simulink model "control_strategy_1"  (R2024b)
settings: Solver=VariableStepAuto  StartTime=0.0  StopTime=0.3  MaxStep=1e-3  MinStep=1e-9  RelTol=1e-3
values from neighbouring files (symbols this model uses):
  C_filtre = 1 / (Lc * (2 * pi * 2000)^2)    (= 2.53302959106e-06)    [acdc_converter_parameters.m]
  Ccb = 330e-6    (= 0.00033)    [dcdc_converter_parameters.m]
  Cdc = 2200e-6    (= 0.0022)    [acdc_converter_parameters.m]
  Ci = 220e-6    (= 0.00022)    [dcdc_converter_parameters.m]
  Is = P / Vac    [acdc_converter_parameters.m]
  KI = KP * Wci_out    [dcdc_converter_main.m]
  KI_curr_d = 2 * pi * w_i * rac    [acdc_converter_main.m]
  KI_curr_q = 2 * pi * w_i * rac    [acdc_converter_main.m]
  KI_q = C_q.Ki    [acdc_converter_main.m]
  KI_volt = C_volt.Ki    [acdc_converter_main.m]
  KP = Wbi_dc / (DCGain_iod * Wci_out)    [dcdc_converter_main.m]
  KP_curr_d = 2 * pi * w_i * Lc    [acdc_converter_main.m]
  KP_curr_q = 2 * pi * w_i * Lc    [acdc_converter_main.m]
  KP_q = C_q.Kp    [acdc_converter_main.m]
  KP_volt = C_volt.Kp    [acdc_converter_main.m]
  Lb = 3e-3    (= 0.003)    [dcdc_converter_parameters.m]
  Lc = 2.5e-3    (= 0.0025)    [acdc_converter_parameters.m]
  Lsi = 105e-6    (= 0.000105)    [dcdc_converter_parameters.m]
  P = 500    [main_control_strategy_1.m]
  phase = 0    [acdc_converter_parameters.m]
  Q = 0    [main_control_strategy_1.m]
  rac = 1e-3    (= 0.001)    [acdc_converter_parameters.m]
  rb = 1e-3    (= 0.001)    [dcdc_converter_parameters.m]
  ro = 270e-3    (= 0.27)    [dcdc_converter_parameters.m]
  rsi = 1e-3    (= 0.001)    [dcdc_converter_parameters.m]
  Vac = 120    [acdc_converter_parameters.m]
  Vb = 48    [dcdc_converter_parameters.m]
  Vdc0 = Vdc    (= 200)    [acdc_converter_parameters.m]
  Vs0 = Vac    (= 120)    [acdc_converter_parameters.m]
  w = 2 * pi * f    (= 376.991118431)    [acdc_converter_parameters.m]
  Zl = w * Lc    (= 0.942477796077)    [acdc_converter_parameters.m]
undefined symbols (not defined in the file or in its folder): q_switch
libraries: spsSeriesRLCBranchLib x6, spsMosfetLib x6, slpidlib x5, spsVoltageMeasurementLib x4, spsMeanLib x4, spsParallelRLCBranchLib x3, spsCurrentMeasurementLib x3, spsTHDLib x3, spsACVoltageSourceLib x1, spsGroundLib x1, spsPWMGenerator2LevelLib x1, eePowerMeasurement x1
settings Model: Creator=casti  LastModifiedBy=Asus
settings OptimizationCC: ReuseModelBlockBuffer=off
settings RTWCC: GPUComputeCapability=3.5

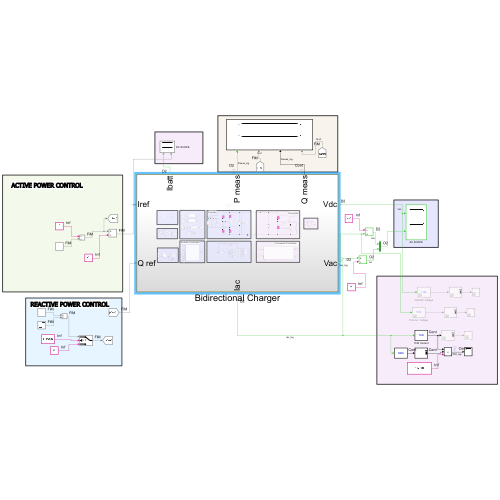
[thumbnail: Simulink's stored preview of the top-level diagram]
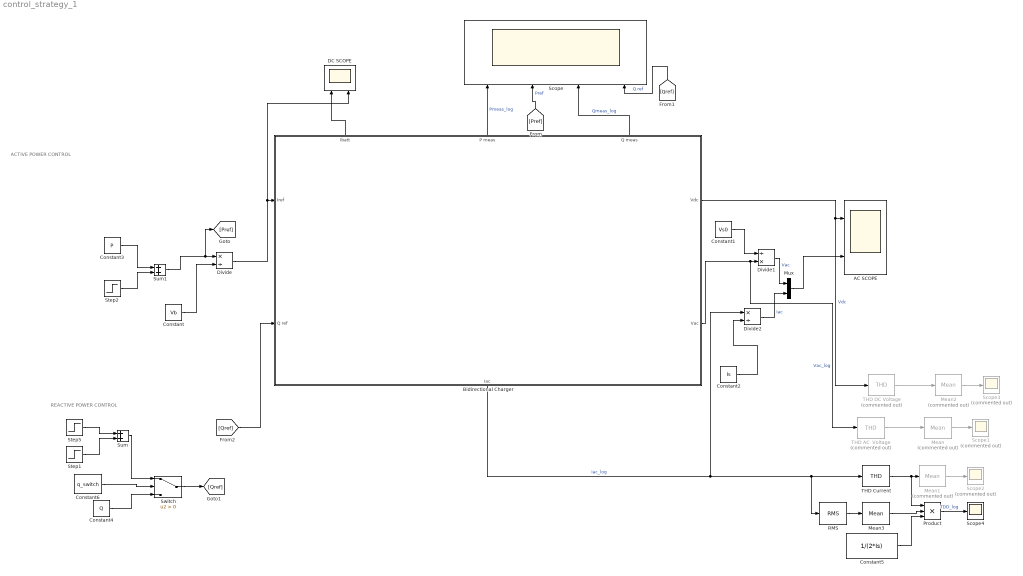
== system control_strategy_1 ==
  note: ACTIVE POWER CONTROL
  note: REACTIVE POWER CONTROL
  AC SCOPE : Scope  NumInputPorts=2
  Bidirectional Charger : Subsystem
      settings: PortSchema="{\"entries\":[{\"content\":{\"sides\":[{\"content\":{\"connectorIds\":[\"In1\",\"In2\"]},\"type\":\"ConnectorPlacement.EquallySpacedRectSide\",\"uuid\":\"0e8ef780-485e-4c8b-9a8b-f034f795c892\"},{\"content\":{\"connectorIds\":[\"Out1\",\"Out2\"],\"side\":\"RIGHT\"},\"type\":\"ConnectorPlacement.EquallySpacedRectSide\",\"uuid\":\"9fd702af-2122-4ac4-9fd2-64e19671b5dd\"},{\"content\":{\"connectorIds\":[\"Out4\",\"Out5\",\"Out6\"],\"side\":\"TOP\"},\"type\":\"ConnectorPlacement.EquallySpacedRectSide\",\"uuid\":\"331bdb16-1cb1-49e4-96bf-e66e7b38baa0\"},{\"content\":{\"connectorIds\":[\"Out3\"],\"side\":\"BOTTOM\"},\"type\":\"ConnectorPlacement.EquallySpacedRectSide\",\"uuid\":\"d0f2bc9b-30cd-4241-b923-1d5d9998130d\"}]},\"type\":\"ConnectorPlacement.EquallySpacedConnector\",\"uuid\":\"78325ce0-b63a-4b2a-b520-d47ca5f2449f\"}],\"packageUris\":[\"http://schema.mathworks.com/mf0/Connector/R2020b\"],\"version\":\"1.0\"}"
  Constant : Constant  Value=Vb
  Constant1 : Constant  Value=Vs0
  Constant2 : Constant  Value=Is
  Constant3 : Constant  Value=P
  Constant4 : Constant  Value=Q
  Constant5 : Constant  Value=1/(2*Is)
  Constant6 : Constant  Value=q_switch
  DC SCOPE : Scope  NumInputPorts=2
  Divide : Product  Inputs=*/
  Divide1 : Product  Inputs=/*
  Divide2 : Product  Inputs=*/
  Mean : spsMeanLib/Mean  Commented=on  Freq=60  Vinit=0  Ts=0
  Mean1 : spsMeanLib/Mean  Commented=on  Freq=60  Vinit=0  Ts=0
  Mean2 : spsMeanLib/Mean  Commented=on  Freq=120  Vinit=0  Ts=0
  Mean3 : spsMeanLib/Mean  Freq=60  Vinit=0  Ts=0
  Mux : Mux  Inputs=2
  Product : Product  Inputs=3
  RMS : spsRMSLib/RMS  TrueRMS=on  Freq=60  RMSInit=120  Ts=0
  Scope : Scope  NumInputPorts=4
  Scope1 : Scope  Commented=on
  Scope2 : Scope  Commented=on
  Scope3 : Scope  Commented=on
  Scope4 : Scope
  Step1 : Step  Time=10  After=-2*Q  SampleTime=0
  Step2 : Step  Time=10  After=-2*P  SampleTime=0
  Step5 : Step  Time=0.05  After=Q  SampleTime=0
  Sum : Sum
  Sum1 : Sum
  Switch : Switch  Criteria=u2 > Threshold  SaturateOnIntegerOverflow=off  InputSameDT=off
  THD AC  Voltage : spsTHDLib/THD  Commented=on  Freq=60  Ts=0
  THD Current : spsTHDLib/THD  Freq=60  Ts=0
  THD DC Voltage : spsTHDLib/THD  Commented=on  Freq=120  Ts=0
  wires:
  Constant/1 -> Divide/2
  Divide/1 -> DC SCOPE/2, Bidirectional Charger/1(Iref)
  Bidirectional Charger/4(Ibatt) -> DC SCOPE/1
  Bidirectional Charger/1(Vdc) -> THD DC Voltage/1, AC SCOPE/1  "Vdc"
  Bidirectional Charger/5(P meas) -> Scope/1  "Pmeas_log"
  Bidirectional Charger/6(Q meas) -> Scope/3  "Qmeas_log"
  [Pref] -> Scope/2  "Pref"
  [Qref] -> Scope/4  "Q ref"
  Mux/1 -> AC SCOPE/2
  Bidirectional Charger/2(Vac) -> THD AC  Voltage/1, Divide1/2  "Vac_log"
  Constant1/1 -> Divide1/1
  Constant2/1 -> Divide2/2
  Divide2/1 -> Mux/2  "Iac"
  Divide1/1 -> Mux/1  "Vac"
  Mean/1 -> Scope1/1
  THD AC  Voltage/1 -> Mean/1
  Mean1/1 -> Scope2/1
  THD Current/1 -> Product/1, Mean1/1
  THD DC Voltage/1 -> Mean2/1
  Mean2/1 -> Scope3/1
  [Qref] -> Bidirectional Charger/2(Q ref)
  RMS/1 -> Mean3/1
  Constant5/1 -> Product/3
  Product/1 -> Scope4/1  "TDD_log"
  Mean3/1 -> Product/2
  Bidirectional Charger/3(Iac) -> RMS/1, THD Current/1, Divide2/1  "Iac_log"
  Constant4/1 -> Switch/3
  Switch/1 -> [Qref]
  Constant6/1 -> Switch/2
  Step5/1 -> Sum/1
  Sum/1 -> Switch/1
  Step1/1 -> Sum/2
  Step2/1 -> Sum1/2
  Constant3/1 -> Sum1/1
  Sum1/1 -> [Pref], Divide/1

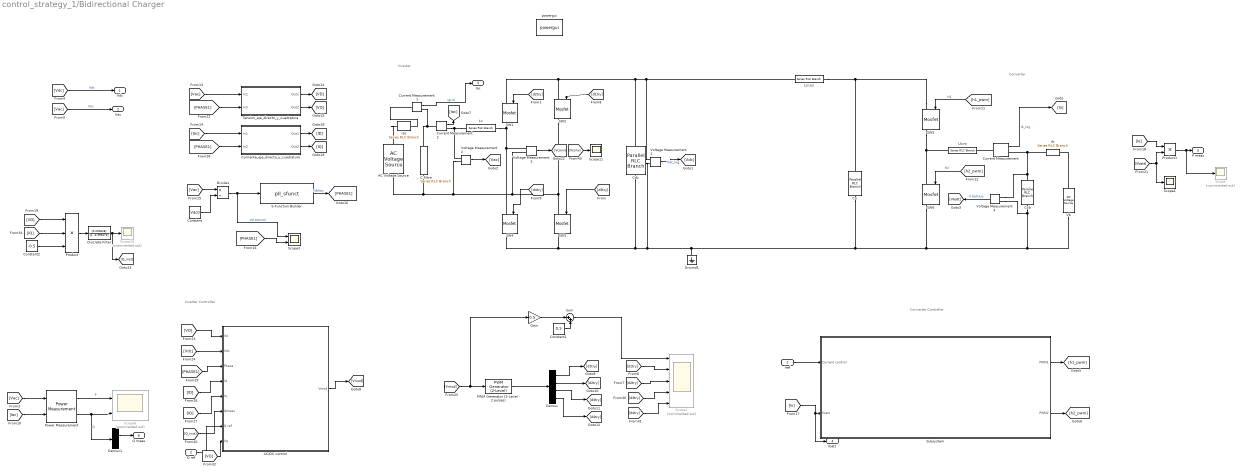
== system control_strategy_1/Bidirectional Charger ==
  note: Converter
  note: Inverter Controller
  note: Inverter
  note: Converter Controller
  Iref : Inport
  Q ref : Inport  Port=2
  AC Voltage Source : spsACVoltageSourceLib/AC Voltage Source  Amplitude=Vac*sqrt(2)  Phase=0  Frequency=60  SampleTime=0  Measurements=None  BusType=swing  Pref=10e3  Qref=0  Qmin=-inf  Qmax=+inf
  AC/DC control : Subsystem
  C filtre : spsSeriesRLCBranchLib/Series RLC Branch  LConnTagsString=__new0  RConnTagsString=__new0  BranchType=C  Resistance=rac  Inductance=Lc  SetiL0=off  InitialCurrent=Io0  Capacitance=C_filtre  Setx0=off  InitialVoltage=0  Measurements=None
  Ccb : spsParallelRLCBranchLib/Parallel RLC Branch  LConnTagsString=a  RConnTagsString=__new0  BranchType=C  Resistance=1  Inductance=1e-3  SetiL0=off  InitialCurrent=0  Capacitance=Ccb  Setx0=on  InitialVoltage=Vb  Measurements=None
  Cdc : spsParallelRLCBranchLib/Parallel RLC Branch  LConnTagsString=a  RConnTagsString=__new0  BranchType=C  Resistance=1  Inductance=1e-3  SetiL0=off  InitialCurrent=0  Capacitance=Cdc  Setx0=on  InitialVoltage=Vdc  Measurements=None
  Constant : Constant  Value=Vdc0
  Constant1 : Constant  Value=0.5
  Constant2 : Constant  Value=-0.5
  Corriente_eje_directo_y_cuadratura : Subsystem
  Csi : spsParallelRLCBranchLib/Parallel RLC Branch  LConnTagsString=a  RConnTagsString=__new0  BranchType=C  Resistance=1  Inductance=1e-3  SetiL0=off  InitialCurrent=0  Capacitance=Ci  Setx0=on  InitialVoltage=Vdc  Measurements=None
  Current Measurement : spsCurrentMeasurementLib/Current Measurement  PhasorSimulation=off  OutputType=Complex  PSBequivalent=0
  Current Measurement1 : spsCurrentMeasurementLib/Current Measurement  PhasorSimulation=off  OutputType=Complex  PSBequivalent=0
  Current Measurement2 : spsCurrentMeasurementLib/Current Measurement  PhasorSimulation=off  OutputType=Complex  PSBequivalent=0
  Demux : Demux
  Demux1 : Demux
  Discrete Filter : DiscreteFilter  Numerator=[0.000628]  Denominator=[1 -0.999372]
  Divide1 : Product  Inputs=*/
  Gain : Gain  Gain=0.5
  Ground1 : spsGroundLib/Ground  LConnTagsString=a
  Lb,ro : spsSeriesRLCBranchLib/Series RLC Branch  LConnTagsString=__new0  RConnTagsString=__new0  BranchType=RL  Resistance=ro  Inductance=Lb  SetiL0=off  InitialCurrent=Io0  Capacitance=1e-6  Setx0=off  InitialVoltage=0  Measurements=None
  Lc : spsSeriesRLCBranchLib/Series RLC Branch  LConnTagsString=__new0  RConnTagsString=__new0  BranchType=L  Resistance=rac  Inductance=Lc  SetiL0=off  InitialCurrent=Io0  Capacitance=1e-6  Setx0=off  InitialVoltage=0  Measurements=None
  Lsi,rsi : spsSeriesRLCBranchLib/Series RLC Branch  LConnTagsString=__new0  RConnTagsString=__new0  BranchType=RL  Resistance=rsi  Inductance=Lsi  SetiL0=off  InitialCurrent=Io0  Capacitance=1e-6  Setx0=off  InitialVoltage=0  Measurements=None
  PWM Generator (2-Level - 2 pulses) : spsPWMGenerator2LevelLib/PWM Generator (2-Level)  ModulatorType=Single-phase full-bridge - Bipolar modulation (4 pulses)  ModulatorMode=Unsynchronized  Fc=20000  Pc=90  nF=27  MinMax="[ -1  1 ]"  SamplingTechnique=Natural  ModulatingSignals=off  m=0.6  Freq=60  Phase=30  Ts=5e-6  ShowCarrierOutport=off
  Power Measurement : eePowerMeasurement/Power Measurement  LabelModeActiveChoice=Continuous  F=60  K=[0 1 2 3]  Ts=0
  Product : Product  Inputs=3
  Product1 : Product
  S-Function Builder : S-Function  FunctionName=pll_sfunct  SFunctionModules=pll_sfunct_wrapper.c  SFunctionDeploymentMode=off  EnableBusSupport=off  mask(S-Function Builder){}
      mask help: Simulink:masks:SFunctionBuilder_MD
      mask init:
      | val = [[.9  0.75 0.75 1 1 .9 .9 1]',[1 1 0.75 0.75 .9 .9 1 .9]'];try , sys = get_param(gcb,'SfunBuilderFcnName');if isempty(sys), sys = get_param(gcb,'FunctionName'); end,catch, sys = get_param(gcb,'FunctionName'); end
      settings: CopyFcn=set_param(gcbh,'LinkStatus','none')  OpenFcn=sfunctionwizard(gcbh)
      mask Display:
      | plot(val(:,1),val(:,2))
      | disp(sys)
      | port_label('input',1,sprintf('%s', 'Vac'),'interpreter','tex')
      | port_label('output',1,sprintf('%s', 'phase'),'interpreter','tex')
  SW{1..6} (6 alike) : spsMosfetLib/Mosfet  Ron=1e-3  Lon=0  Rd=0.00001  Vfd=0  IC=0  Rs=1e5  Cs=inf  Measurements=on
  Scope : Scope  Commented=on
  Scope1 : Scope
  Scope10 : Scope  Commented=on
  Scope11 : Scope
  Scope2 : Scope  Commented=on  NumInputPorts=5
  Scope3 : Scope  NumInputPorts=2
  Scope8 : Scope  Commented=on  NumInputPorts=2
  Subsystem : Subsystem
  Sum : Sum  Inputs=|++
  Tension_eje_directo_y_cuadratura : Subsystem
  Vb : spsDCVoltageSourceLib/DC Voltage Source  Amplitude=Vb  Measurements=None
  Voltage Measurement{1..4} (4 alike) : spsVoltageMeasurementLib/Voltage Measurement  PhasorSimulation=off  OutputType=Complex  PSBequivalent=0
  powergui : spspowerguiLib/powergui  Priority=1  SimulationMode=Discrete  SampleTime=5e-6  frequency=60  Iterations=50  frequencyindice=0  Pbase=100e6  ErrMax=1e-4  UnitsV=kV  UnitsW=MW  buscounter=0  FunctionMessages=off  echomessages=off  EnableUseOfTLC=off  CurrentSourceSwitches=off  DisableSnubberDevices=off  DisableRonSwitches=off  DisableVfSwitches=off  DisplayEquations=off  AutomaticDiscreteSolvers=off  SolverType=Tustin/Backward Euler (TBE)  Interpol=off  ExternalGateDelay=off  methode=off  Ts=100  x0status=blocks  SPID=on  SwTol=0  HookPort=off  NonlinearTolerance=1e-4  nMaxIteration=100  ContinueOnMaxIteration=off  RestoreLinks=warning  ResistiveCurrentMeasurement=off  Frange=[0:2:500]  Ylog=off  Xlog=on  ShowGrid=off  save=off  variable=ZData  structure=0  ZoomFFT=off  StartTime=0.0  cycles=1  DisplayStyle=1  fundamental=60  FreqAxis=off  MaxFrequency=1000  frequencyindicesteady=1  RmsSteady=1  display=off
  rac : spsSeriesRLCBranchLib/Series RLC Branch  LConnTagsString=__new0  RConnTagsString=__new0  BranchType=R  Resistance=rac  Inductance=Lc  SetiL0=off  InitialCurrent=Io0  Capacitance=1e-6  Setx0=off  InitialVoltage=0  Measurements=None
  rb : spsSeriesRLCBranchLib/Series RLC Branch  LConnTagsString=__new0  RConnTagsString=__new0  BranchType=R  Resistance=rb  Inductance=1e-3  SetiL0=off  InitialCurrent=0  Capacitance=1e-6  Setx0=off  InitialVoltage=0  Measurements=None
  Vdc : Outport
  Vac : Outport  Port=2
  Iac : Outport  Port=3
  Ibatt : Outport  Port=4
  P meas : Outport  Port=5
  Q meas : Outport  Port=6
  wires:
  Iref/1 -> Subsystem/1(Current control)
  [d2try] -> Scope2/3
  Voltage Measurement3/1 -> [Vconv]
  PWM Generator (2-Level - 2 pulses)/1 -> Demux/1
  [Vconv] -> Scope11/1
  [Io] -> Ibatt/1, Subsystem/2(Ibatt)
  [PHASE1] -> Corriente_eje_directo_y_cuadratura/2(In2)
  [h1_pwm] -> SW5/1  "H1"
  [Vac] -> Vac/1  "Vac"
  [Vac] -> Divide1/1
  AC/DC control/1(Vmod) -> [Vmod]
  Tension_eje_directo_y_cuadratura/1(Out1) -> [VD]
  Gain/1 -> Sum/1
  [Iac] -> Corriente_eje_directo_y_cuadratura/1(In1)
  Divide1/1 -> Scope3/1, S-Function Builder/1  "Vd control"
  Sum/1 -> Scope2/1
  [h2_pwm] -> SW6/1  "H2"
  Current Measurement2/1 -> [Iac]
  Subsystem/2(PWM2) -> [h2_pwm]
  Voltage Measurement1/1 -> [Vdc]  "Vdc_log"
  Current Measurement/1 -> [Io]  "Ib_log"
  [d2try] -> SW1/1
  Demux/4 -> [d4try]
  Constant1/1 -> Sum/2
  [Vdc] -> Vdc/1  "Vdc"
  [d1try] -> SW2/1
  Constant/1 -> Divide1/2
  [d4try] -> Scope2/5
  [d3try] -> SW3/1
  S-Function Builder/1 -> [PHASE1]  "Vdelay"
  Voltage Measurement2/1 -> [Vac]
  Demux/1 -> [d1try]
  [Vmod] -> Gain/1, PWM Generator (2-Level - 2 pulses)/1
  [d4try] -> SW4/1
  Subsystem/1(PWM1) -> [h1_pwm]
  [Vac] -> Tension_eje_directo_y_cuadratura/1(In1)
  Tension_eje_directo_y_cuadratura/2(Out2) -> [VQ]
  Corriente_eje_directo_y_cuadratura/1(Out1) -> [ID]
  Corriente_eje_directo_y_cuadratura/2(Out2) -> [IQ]
  [PHASE1] -> Scope3/2
  [PHASE1] -> Tension_eje_directo_y_cuadratura/2(In2)
  [ID] -> AC/DC control/4(Id)
  Demux/2 -> [d2try]
  Demux/3 -> [d3try]
  [d3try] -> Scope2/4
  [d1try] -> Scope2/2
  [Vdc] -> AC/DC control/2(Vdc)
  [VD] -> AC/DC control/1(Vd)
  [IQ] -> AC/DC control/5(Iq)
  [PHASE1] -> AC/DC control/3(Phase)
  Power Measurement/2 -> Demux1/1, Scope8/2  "Q"
  [Iac] -> Power Measurement/2
  Demux1/2 -> Q meas/1
  Power Measurement/1 -> Scope8/1  "P"
  [Vac] -> Power Measurement/1
  [Q_inst] -> AC/DC control/6(Qmeas)
  [VD] -> Product/1
  Discrete Filter/1 -> [Q_inst], Scope10/1
  Product/1 -> Discrete Filter/1
  [IQ] -> Product/2
  Constant2/1 -> Product/3
  Q ref/1 -> AC/DC control/7(Q ref)
  Voltage Measurement4/1 -> [Vbatt]  "V battery"
  [Io] -> Product1/1
  [Vbatt] -> Scope1/1, Product1/2
  Product1/1 -> Scope/1, P meas/1
  Current Measurement1/1 -> Iac/1  "igrid"
  [VQ] -> AC/DC control/8(Vq)
  connections:
  SW4/LConn1 -- Lc/RConn1 -- SW1/RConn1 -- Voltage Measurement3/LConn1
  SW5/LConn1 -- Csi/LConn1 -- Lsi,rsi/LConn1
  SW2/LConn1 -- Cdc/LConn1 -- Voltage Measurement1/LConn1 -- Lsi,rsi/RConn1 -- SW1/LConn1
  SW6/RConn1 -- Voltage Measurement4/LConn2 -- Ccb/RConn1 -- Vb/LConn1 -- Csi/RConn1 -- Cdc/RConn1 -- SW3/RConn1 -- SW4/RConn1 -- Voltage Measurement1/LConn2 -- Ground1/LConn1
  Vb/RConn1 -- rb/RConn1
  SW5/RConn1 -- SW6/LConn1 -- Lb,ro/LConn1
  C filtre/LConn1 -- Current Measurement1/RConn1 -- Current Measurement2/LConn1
  Voltage Measurement2/LConn2 -- AC Voltage Source/LConn1 -- C filtre/RConn1 -- SW2/RConn1 -- SW3/LConn1 -- Voltage Measurement3/LConn2
  Ccb/LConn1 -- rb/LConn1 -- Current Measurement/RConn1 -- Voltage Measurement4/LConn1
  Current Measurement/LConn1 -- Lb,ro/RConn1
  Lc/LConn1 -- Current Measurement2/RConn1 -- Voltage Measurement2/LConn1
  rac/RConn1 -- AC Voltage Source/RConn1
  Current Measurement1/LConn1 -- rac/LConn1

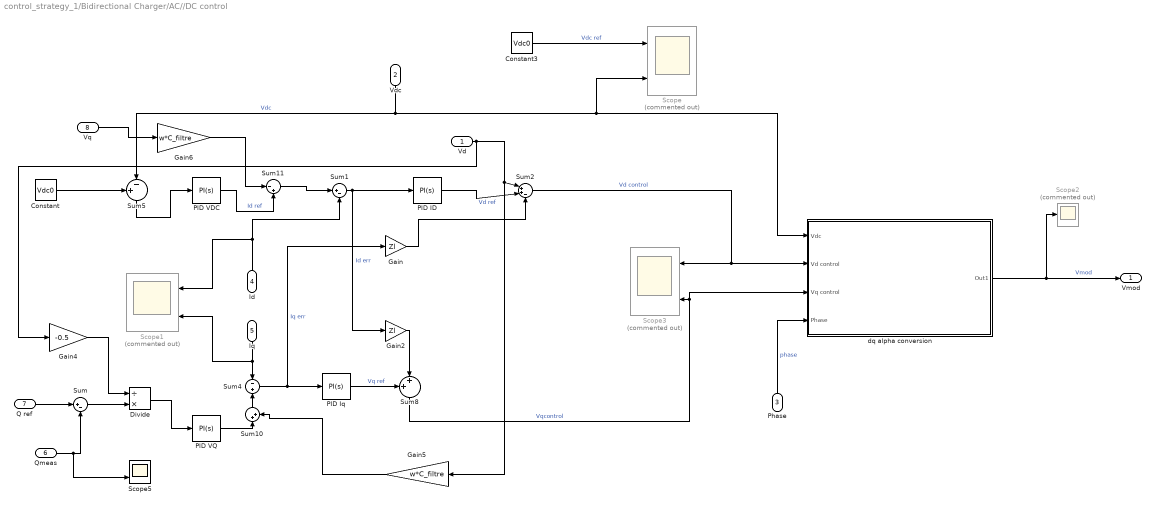
== system control_strategy_1/Bidirectional Charger/AC//DC control ==
  Vd : Inport
  Vdc : Inport  Port=2
  Phase : Inport  Port=3
  Id : Inport  Port=4
  Iq : Inport  Port=5
  Qmeas : Inport  Port=6
  Q ref : Inport  Port=7
  Vq : Inport  Port=8
  Constant : Constant  Value=Vdc0
  Constant3 : Constant  Value=Vdc0
  Divide : Product  Inputs=/*
  Gain : Gain  Gain=Zl
  Gain2 : Gain  Gain=Zl
  Gain4 : Gain  Gain=-0.5
  Gain5 : Gain  Gain=w*C_filtre
  Gain6 : Gain  Gain=w*C_filtre
  PID ID : slpidlib/PID Controller  Controller=PI  Form=Parallel  TimeDomain=Continuous-time  UseExternalTs=off  SampleTime=-1  IntegratorMethod=Forward Euler  FilterMethod=Forward Euler  ControllerParametersSource=internal  P=KP_curr_d  I=KI_curr_d  UseKiTs=off  D=0  UseExternalDerivativeSource=off  N=100  UseFilter=on  TunerSelectOption=Transfer Function Based (PID Tuner App)  InitialConditionSource=internal  InitialConditionForIntegrator=0  InitialConditionForFilter=0  DifferentiatorICPrevScaledInput=0  ExternalReset=none  TrackingMode=off  Kt=1  LimitOutput=off  SatLimitsSource=internal  UpperSaturationLimit=200  LowerSaturationLimit=-inf  LinearizeAsGain=on  AntiWindupMode=none  Kb=1  LimitIntegrator=off  UpperIntegratorSaturationLimit=inf  LowerIntegratorSaturationLimit=-inf  POutMin=[]  POutMax=[]  IOutMin=[]  IOutMax=[]  DOutMin=[]  DOutMax=[]  NOutMin=[]  NOutMax=[]  SumOutMin=[]  SumOutMax=[]  SaturationOutMin=[]  SaturationOutMax=[]  PParamMin=[]  PParamMax=[]  IParamMin=[]  IParamMax=[]  DParamMin=[]  DParamMax=[]  NParamMin=[]  NParamMax=[]  KbParamMin=[]  KbParamMax=[]  KtParamMin=[]  KtParamMax=[]  KbOutMin=[]  KbOutMax=[]  KtOutMin=[]  KtOutMax=[]  IntegratorOutMin=[]  IntegratorOutMax=[]  FilterOutMin=[]  FilterOutMax=[]  SumI1OutMin=[]  SumI1OutMax=[]  SumI2OutMin=[]  SumI2OutMax=[]  SumI3OutMin=[]  SumI3OutMax=[]  SumI4OutMin=[]  SumI4OutMax=[]  SumDOutMin=[]  SumDOutMax=[]  DifferentiatorOutMin=[]  DifferentiatorOutMax=[]  FilterDiffOutCoefMin=[]  FilterDiffOutCoefMax=[]  ReciprocalOutMin=[]  ReciprocalOutMax=[]  SumDenOutMin=[]  SumDenOutMax=[]  SumNumOutMin=[]  SumNumOutMax=[]  DivideOutMin=[]  DivideOutMax=[]  UdiffTsProdOutMin=[]  UdiffTsProdOutMax=[]  NTsProdOutMin=[]  NTsProdOutMax=[]  UintegralTsProdOutMin=[]  UintegralTsProdOutMax=[]  UngainTsProdOutMin=[]  UngainTsProdOutMax=[]  ClampingZeroOutDataTypeStr=Inherit: Inherit via back propagation  ClampingZeroOutMin=[]  ClampingZeroOutMax=[]  FilterDenConstantOutDataTypeStr=Inherit: Inherit via back propagation  FilterDenConstantOutMin=[]  FilterDenConstantOutMax=[]  PCopyOutDataTypeStr=Inherit: Inherit via back propagation  PCopyOutMin=[]  PCopyOutMax=[]  NCopyOutDataTypeStr=Inherit: Inherit via back propagation  NCopyOutMin=[]  NCopyOutMax=[]  IntegratorContinuousStateAttributes=''  IntegratorStateMustResolveToSignalObject=off  IntegratorRTWStateStorageClass=Auto  FilterContinuousStateAttributes=''  FilterStateMustResolveToSignalObject=off  FilterRTWStateStorageClass=Auto  ParallelPVariant=InternalParameters  IdealPVariant=Disabled  IVariant=InternalParameters  DVariant=Disabled  IntegratorVariant=Continuous  SatVariant=Disabled  AWVariant=Passthrough  PCopyVariant=Disabled  TRVariant=Disabled  FdbkBlocksVariant=Forward  IdealPFdbkVariant=Disabled  SatFdbkVariant=Disabled  DerivativeFilterVariant=Disabled  NVariant=Disabled  NCopyVariant=Disabled_SignalSpec  FilterICVariant=Disabled  IntegratorICVariant=InternalICs  ExternalResetVariant=Disabled  TRSumVariant=Passthrough  SumFdbkVariant=Disabled  SumVariant=Sum_PI  TsampFilterVariant=InternalTs  TsampNgainVariant=Passthrough  TsampIntegralVariant=Disabled_SignalSpec  ExternalSaturationOutDataTypeStr=Inherit: Same as second input  DerivativeSourceVariant=Disabled  PreIntVariant=InternalPreInt
  PID Iq : slpidlib/PID Controller  Controller=PI  Form=Parallel  TimeDomain=Continuous-time  UseExternalTs=off  SampleTime=-1  IntegratorMethod=Forward Euler  FilterMethod=Forward Euler  ControllerParametersSource=internal  P=KP_curr_q  I=KI_curr_q  UseKiTs=off  D=0  UseExternalDerivativeSource=off  N=100  UseFilter=on  TunerSelectOption=Transfer Function Based (PID Tuner App)  InitialConditionSource=internal  InitialConditionForIntegrator=0  InitialConditionForFilter=0  DifferentiatorICPrevScaledInput=0  ExternalReset=none  TrackingMode=off  Kt=1  LimitOutput=off  SatLimitsSource=internal  UpperSaturationLimit=15  LowerSaturationLimit=-15  LinearizeAsGain=on  AntiWindupMode=none  Kb=1  LimitIntegrator=off  UpperIntegratorSaturationLimit=inf  LowerIntegratorSaturationLimit=-inf  POutMin=[]  POutMax=[]  IOutMin=[]  IOutMax=[]  DOutMin=[]  DOutMax=[]  NOutMin=[]  NOutMax=[]  SumOutMin=[]  SumOutMax=[]  SaturationOutMin=[]  SaturationOutMax=[]  PParamMin=[]  PParamMax=[]  IParamMin=[]  IParamMax=[]  DParamMin=[]  DParamMax=[]  NParamMin=[]  NParamMax=[]  KbParamMin=[]  KbParamMax=[]  KtParamMin=[]  KtParamMax=[]  KbOutMin=[]  KbOutMax=[]  KtOutMin=[]  KtOutMax=[]  IntegratorOutMin=[]  IntegratorOutMax=[]  FilterOutMin=[]  FilterOutMax=[]  SumI1OutMin=[]  SumI1OutMax=[]  SumI2OutMin=[]  SumI2OutMax=[]  SumI3OutMin=[]  SumI3OutMax=[]  SumI4OutMin=[]  SumI4OutMax=[]  SumDOutMin=[]  SumDOutMax=[]  DifferentiatorOutMin=[]  DifferentiatorOutMax=[]  FilterDiffOutCoefMin=[]  FilterDiffOutCoefMax=[]  ReciprocalOutMin=[]  ReciprocalOutMax=[]  SumDenOutMin=[]  SumDenOutMax=[]  SumNumOutMin=[]  SumNumOutMax=[]  DivideOutMin=[]  DivideOutMax=[]  UdiffTsProdOutMin=[]  UdiffTsProdOutMax=[]  NTsProdOutMin=[]  NTsProdOutMax=[]  UintegralTsProdOutMin=[]  UintegralTsProdOutMax=[]  UngainTsProdOutMin=[]  UngainTsProdOutMax=[]  ClampingZeroOutDataTypeStr=Inherit: Inherit via back propagation  ClampingZeroOutMin=[]  ClampingZeroOutMax=[]  FilterDenConstantOutDataTypeStr=Inherit: Inherit via back propagation  FilterDenConstantOutMin=[]  FilterDenConstantOutMax=[]  PCopyOutDataTypeStr=Inherit: Inherit via back propagation  PCopyOutMin=[]  PCopyOutMax=[]  NCopyOutDataTypeStr=Inherit: Inherit via back propagation  NCopyOutMin=[]  NCopyOutMax=[]  IntegratorContinuousStateAttributes=''  IntegratorStateMustResolveToSignalObject=off  IntegratorRTWStateStorageClass=Auto  FilterContinuousStateAttributes=''  FilterStateMustResolveToSignalObject=off  FilterRTWStateStorageClass=Auto  ParallelPVariant=InternalParameters  IdealPVariant=Disabled  IVariant=InternalParameters  DVariant=Disabled  IntegratorVariant=Continuous  SatVariant=Disabled  AWVariant=Passthrough  PCopyVariant=Disabled  TRVariant=Disabled  FdbkBlocksVariant=Forward  IdealPFdbkVariant=Disabled  SatFdbkVariant=Disabled  DerivativeFilterVariant=Disabled  NVariant=Disabled  NCopyVariant=Disabled_SignalSpec  FilterICVariant=Disabled  IntegratorICVariant=InternalICs  ExternalResetVariant=Disabled  TRSumVariant=Passthrough  SumFdbkVariant=Disabled  SumVariant=Sum_PI  TsampFilterVariant=InternalTs  TsampNgainVariant=Passthrough  TsampIntegralVariant=Disabled_SignalSpec  ExternalSaturationOutDataTypeStr=Inherit: Same as second input  DerivativeSourceVariant=Disabled  PreIntVariant=InternalPreInt
  PID VDC : slpidlib/PID Controller  Controller=PI  Form=Parallel  TimeDomain=Continuous-time  UseExternalTs=off  SampleTime=-1  IntegratorMethod=Forward Euler  FilterMethod=Forward Euler  ControllerParametersSource=internal  P=-KP_volt  I=-KI_volt  UseKiTs=off  D=0  UseExternalDerivativeSource=off  N=100  UseFilter=on  TunerSelectOption=Frequency Response Based  InitialConditionSource=internal  InitialConditionForIntegrator=0  InitialConditionForFilter=0  DifferentiatorICPrevScaledInput=0  ExternalReset=none  TrackingMode=off  Kt=1  LimitOutput=off  SatLimitsSource=internal  UpperSaturationLimit=16  LowerSaturationLimit=-16  LinearizeAsGain=on  AntiWindupMode=none  Kb=1  LimitIntegrator=off  UpperIntegratorSaturationLimit=inf  LowerIntegratorSaturationLimit=-inf  POutMin=[]  POutMax=[]  IOutMin=[]  IOutMax=[]  DOutMin=[]  DOutMax=[]  NOutMin=[]  NOutMax=[]  SumOutMin=[]  SumOutMax=[]  SaturationOutMin=[]  SaturationOutMax=[]  PParamMin=[]  PParamMax=[]  IParamMin=[]  IParamMax=[]  DParamMin=[]  DParamMax=[]  NParamMin=[]  NParamMax=[]  KbParamMin=[]  KbParamMax=[]  KtParamMin=[]  KtParamMax=[]  KbOutMin=[]  KbOutMax=[]  KtOutMin=[]  KtOutMax=[]  IntegratorOutMin=[]  IntegratorOutMax=[]  FilterOutMin=[]  FilterOutMax=[]  SumI1OutMin=[]  SumI1OutMax=[]  SumI2OutMin=[]  SumI2OutMax=[]  SumI3OutMin=[]  SumI3OutMax=[]  SumI4OutMin=[]  SumI4OutMax=[]  SumDOutMin=[]  SumDOutMax=[]  DifferentiatorOutMin=[]  DifferentiatorOutMax=[]  FilterDiffOutCoefMin=[]  FilterDiffOutCoefMax=[]  ReciprocalOutMin=[]  ReciprocalOutMax=[]  SumDenOutMin=[]  SumDenOutMax=[]  SumNumOutMin=[]  SumNumOutMax=[]  DivideOutMin=[]  DivideOutMax=[]  UdiffTsProdOutMin=[]  UdiffTsProdOutMax=[]  NTsProdOutMin=[]  NTsProdOutMax=[]  UintegralTsProdOutMin=[]  UintegralTsProdOutMax=[]  UngainTsProdOutMin=[]  UngainTsProdOutMax=[]  ClampingZeroOutDataTypeStr=Inherit: Inherit via back propagation  ClampingZeroOutMin=[]  ClampingZeroOutMax=[]  FilterDenConstantOutDataTypeStr=Inherit: Inherit via back propagation  FilterDenConstantOutMin=[]  FilterDenConstantOutMax=[]  PCopyOutDataTypeStr=Inherit: Inherit via back propagation  PCopyOutMin=[]  PCopyOutMax=[]  NCopyOutDataTypeStr=Inherit: Inherit via back propagation  NCopyOutMin=[]  NCopyOutMax=[]  IntegratorContinuousStateAttributes=''  IntegratorStateMustResolveToSignalObject=off  IntegratorRTWStateStorageClass=Auto  FilterContinuousStateAttributes=''  FilterStateMustResolveToSignalObject=off  FilterRTWStateStorageClass=Auto  ParallelPVariant=InternalParameters  IdealPVariant=Disabled  IVariant=InternalParameters  DVariant=Disabled  IntegratorVariant=Continuous  SatVariant=Disabled  AWVariant=Passthrough  PCopyVariant=Disabled  TRVariant=Disabled  FdbkBlocksVariant=Forward  IdealPFdbkVariant=Disabled  SatFdbkVariant=Disabled  DerivativeFilterVariant=Disabled  NVariant=Disabled  NCopyVariant=Disabled_SignalSpec  FilterICVariant=Disabled  IntegratorICVariant=InternalICs  ExternalResetVariant=Disabled  TRSumVariant=Passthrough  SumFdbkVariant=Disabled  SumVariant=Sum_PI  TsampFilterVariant=InternalTs  TsampNgainVariant=Passthrough  TsampIntegralVariant=Disabled_SignalSpec  ExternalSaturationOutDataTypeStr=Inherit: Same as second input  DerivativeSourceVariant=Disabled  PreIntVariant=InternalPreInt
  PID VQ : slpidlib/PID Controller  Controller=PI  Form=Parallel  TimeDomain=Continuous-time  UseExternalTs=off  SampleTime=-1  IntegratorMethod=Forward Euler  FilterMethod=Forward Euler  ControllerParametersSource=internal  P=KP_q  I=KI_q  UseKiTs=off  D=0  UseExternalDerivativeSource=off  N=100  UseFilter=on  TunerSelectOption=Frequency Response Based  InitialConditionSource=internal  InitialConditionForIntegrator=0  InitialConditionForFilter=0  DifferentiatorICPrevScaledInput=0  ExternalReset=none  TrackingMode=off  Kt=1  LimitOutput=off  SatLimitsSource=internal  UpperSaturationLimit=100  LowerSaturationLimit=-100  LinearizeAsGain=on  AntiWindupMode=none  Kb=1  LimitIntegrator=off  UpperIntegratorSaturationLimit=inf  LowerIntegratorSaturationLimit=-inf  POutMin=[]  POutMax=[]  IOutMin=[]  IOutMax=[]  DOutMin=[]  DOutMax=[]  NOutMin=[]  NOutMax=[]  SumOutMin=[]  SumOutMax=[]  SaturationOutMin=[]  SaturationOutMax=[]  PParamMin=[]  PParamMax=[]  IParamMin=[]  IParamMax=[]  DParamMin=[]  DParamMax=[]  NParamMin=[]  NParamMax=[]  KbParamMin=[]  KbParamMax=[]  KtParamMin=[]  KtParamMax=[]  KbOutMin=[]  KbOutMax=[]  KtOutMin=[]  KtOutMax=[]  IntegratorOutMin=[]  IntegratorOutMax=[]  FilterOutMin=[]  FilterOutMax=[]  SumI1OutMin=[]  SumI1OutMax=[]  SumI2OutMin=[]  SumI2OutMax=[]  SumI3OutMin=[]  SumI3OutMax=[]  SumI4OutMin=[]  SumI4OutMax=[]  SumDOutMin=[]  SumDOutMax=[]  DifferentiatorOutMin=[]  DifferentiatorOutMax=[]  FilterDiffOutCoefMin=[]  FilterDiffOutCoefMax=[]  ReciprocalOutMin=[]  ReciprocalOutMax=[]  SumDenOutMin=[]  SumDenOutMax=[]  SumNumOutMin=[]  SumNumOutMax=[]  DivideOutMin=[]  DivideOutMax=[]  UdiffTsProdOutMin=[]  UdiffTsProdOutMax=[]  NTsProdOutMin=[]  NTsProdOutMax=[]  UintegralTsProdOutMin=[]  UintegralTsProdOutMax=[]  UngainTsProdOutMin=[]  UngainTsProdOutMax=[]  ClampingZeroOutDataTypeStr=Inherit: Inherit via back propagation  ClampingZeroOutMin=[]  ClampingZeroOutMax=[]  FilterDenConstantOutDataTypeStr=Inherit: Inherit via back propagation  FilterDenConstantOutMin=[]  FilterDenConstantOutMax=[]  PCopyOutDataTypeStr=Inherit: Inherit via back propagation  PCopyOutMin=[]  PCopyOutMax=[]  NCopyOutDataTypeStr=Inherit: Inherit via back propagation  NCopyOutMin=[]  NCopyOutMax=[]  IntegratorContinuousStateAttributes=''  IntegratorStateMustResolveToSignalObject=off  IntegratorRTWStateStorageClass=Auto  FilterContinuousStateAttributes=''  FilterStateMustResolveToSignalObject=off  FilterRTWStateStorageClass=Auto  ParallelPVariant=InternalParameters  IdealPVariant=Disabled  IVariant=InternalParameters  DVariant=Disabled  IntegratorVariant=Continuous  SatVariant=Disabled  AWVariant=Passthrough  PCopyVariant=Disabled  TRVariant=Disabled  FdbkBlocksVariant=Forward  IdealPFdbkVariant=Disabled  SatFdbkVariant=Disabled  DerivativeFilterVariant=Disabled  NVariant=Disabled  NCopyVariant=Disabled_SignalSpec  FilterICVariant=Disabled  IntegratorICVariant=InternalICs  ExternalResetVariant=Disabled  TRSumVariant=Passthrough  SumFdbkVariant=Disabled  SumVariant=Sum_PI  TsampFilterVariant=InternalTs  TsampNgainVariant=Passthrough  TsampIntegralVariant=Disabled_SignalSpec  ExternalSaturationOutDataTypeStr=Inherit: Same as second input  DerivativeSourceVariant=Disabled  PreIntVariant=InternalPreInt
  Scope : Scope  Commented=on  NumInputPorts=2
  Scope1 : Scope  Commented=on  NumInputPorts=2
  Scope2 : Scope  Commented=on
  Scope3 : Scope  Commented=on  NumInputPorts=2
  Scope5 : Scope  NumInputPorts=2
  Sum : Sum  Inputs=|+-
  Sum1 : Sum  Inputs=|+-
  Sum10 : Sum  Inputs=|++
  Sum11 : Sum  Inputs=|-+
  Sum2 : Sum  Inputs=|++-
  Sum4 : Sum  Inputs=-+
  Sum5 : Sum  Inputs=+-|
  Sum8 : Sum  Inputs=++|
  dq alpha conversion : Subsystem
  Vmod : Outport
  wires:
  Constant/1 -> Sum5/1
  Sum4/1 -> PID Iq/1, Gain/1  "Iq err"
  Sum1/1 -> PID ID/1, Gain2/1  "Id err"
  PID Iq/1 -> Sum8/1  "Vq ref"
  Phase/1 -> dq alpha conversion/4(Phase)  "phase"
  PID ID/1 -> Sum2/2  "Vd ref"
  Vdc/1 -> Scope/2, dq alpha conversion/1(Vdc), Sum5/2  "Vdc"
  dq alpha conversion/1(Out1) -> Scope2/1, Vmod/1  "Vmod"
  Sum5/1 -> PID VDC/1
  Gain/1 -> Sum2/3
  Gain2/1 -> Sum8/2
  Id/1 -> Scope1/1, Sum1/2
  Iq/1 -> Scope1/2, Sum4/1
  Sum2/1 -> Scope3/1, dq alpha conversion/2(Vd control)  "Vd control"
  Sum8/1 -> dq alpha conversion/3(Vq control), Scope3/2  "Vqcontrol"
  Constant3/1 -> Scope/1  "Vdc ref"
  Gain4/1 -> Divide/1
  Divide/1 -> PID VQ/1
  Sum/1 -> Divide/2
  Qmeas/1 -> Scope5/2, Sum/2
  Q ref/1 -> Sum/1
  Vd/1 -> Gain4/1, Gain5/1, Sum2/1
  Gain5/1 -> Sum10/2
  Sum10/1 -> Sum4/2
  PID VQ/1 -> Sum10/1
  Vq/1 -> Gain6/1
  PID VDC/1 -> Sum11/2  "Id ref"
  Sum11/1 -> Sum1/1
  Gain6/1 -> Sum11/1

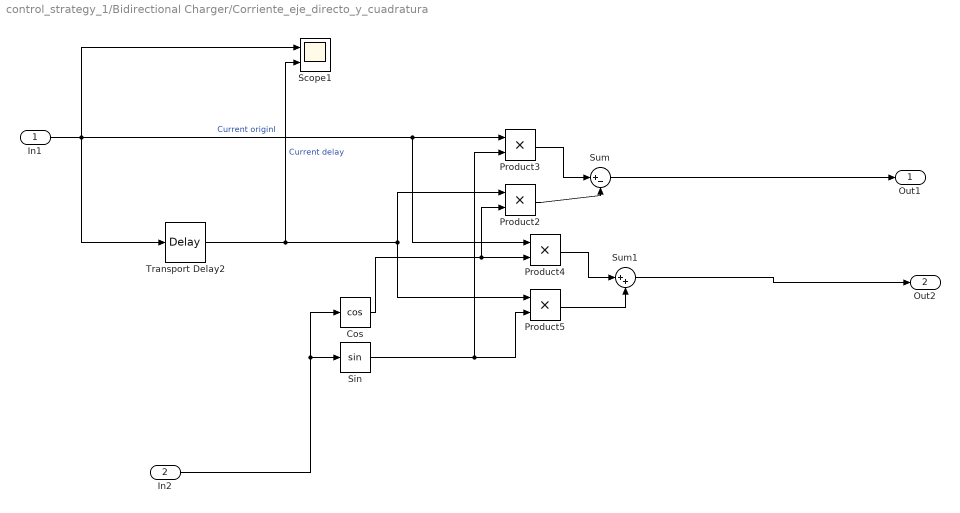
== system control_strategy_1/Bidirectional Charger/Corriente_eje_directo_y_cuadratura ==
  In1 : Inport
  In2 : Inport  Port=2
  Cos : Trigonometry  Operator=cos
  Product{2..5} (4 alike) : Product
  Scope1 : Scope  NumInputPorts=2
  Sin : Trigonometry
  Sum : Sum  Inputs=|+-
  Sum1 : Sum  Inputs=|++
  Transport Delay2 : TransportDelay  DelayTime=0.25/60
  Out1 : Outport
  Out2 : Outport  Port=2
  wires:
  In2/1 -> Sin/1, Cos/1
  Product4/1 -> Sum1/1
  Product3/1 -> Sum/1
  Product5/1 -> Sum1/2
  Sin/1 -> Product5/2, Product3/2
  Sum/1 -> Out1/1
  Sum1/1 -> Out2/1
  In1/1 -> Transport Delay2/1, Product3/1, Product4/1, Scope1/1  "Current originl"
  Transport Delay2/1 -> Scope1/2, Product5/1, Product2/1  "Current delay"
  Cos/1 -> Product2/2, Product4/2
  Product2/1 -> Sum/2

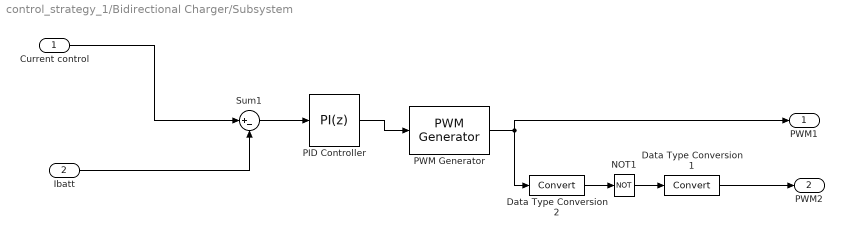
== system control_strategy_1/Bidirectional Charger/Subsystem ==
  Current control : Inport
  Ibatt : Inport  Port=2
  Data Type Conversion1 : DataTypeConversion  SaturateOnIntegerOverflow=off  RndMeth=Floor
  Data Type Conversion2 : DataTypeConversion  SaturateOnIntegerOverflow=off  RndMeth=Floor
  NOT1 : Logic  Operator=NOT  IconShape=distinctive  AllPortsSameDT=off  OutDataTypeStr=boolean
  PID Controller : slpidlib/PID Controller  Controller=PI  Form=Parallel  TimeDomain=Discrete-time  UseExternalTs=off  SampleTime=-1  IntegratorMethod=Forward Euler  FilterMethod=Forward Euler  ControllerParametersSource=internal  P=KP  I=KI  UseKiTs=off  D=0  UseExternalDerivativeSource=off  N=100  UseFilter=on  TunerSelectOption=Transfer Function Based (PID Tuner App)  InitialConditionSource=internal  InitialConditionForIntegrator=0  InitialConditionForFilter=0  DifferentiatorICPrevScaledInput=0  ExternalReset=none  TrackingMode=off  Kt=1  LimitOutput=on  SatLimitsSource=internal  UpperSaturationLimit=1  LowerSaturationLimit=0  LinearizeAsGain=on  AntiWindupMode=none  Kb=1  LimitIntegrator=off  UpperIntegratorSaturationLimit=inf  LowerIntegratorSaturationLimit=-inf  POutMin=[]  POutMax=[]  IOutMin=[]  IOutMax=[]  DOutMin=[]  DOutMax=[]  NOutMin=[]  NOutMax=[]  SumOutMin=[]  SumOutMax=[]  SaturationOutMin=[]  SaturationOutMax=[]  PParamMin=[]  PParamMax=[]  IParamMin=[]  IParamMax=[]  DParamMin=[]  DParamMax=[]  NParamMin=[]  NParamMax=[]  KbParamMin=[]  KbParamMax=[]  KtParamMin=[]  KtParamMax=[]  KbOutMin=[]  KbOutMax=[]  KtOutMin=[]  KtOutMax=[]  IntegratorOutMin=[]  IntegratorOutMax=[]  FilterOutMin=[]  FilterOutMax=[]  SumI1OutMin=[]  SumI1OutMax=[]  SumI2OutMin=[]  SumI2OutMax=[]  SumI3OutMin=[]  SumI3OutMax=[]  SumI4OutMin=[]  SumI4OutMax=[]  SumDOutMin=[]  SumDOutMax=[]  DifferentiatorOutMin=[]  DifferentiatorOutMax=[]  FilterDiffOutCoefMin=[]  FilterDiffOutCoefMax=[]  ReciprocalOutMin=[]  ReciprocalOutMax=[]  SumDenOutMin=[]  SumDenOutMax=[]  SumNumOutMin=[]  SumNumOutMax=[]  DivideOutMin=[]  DivideOutMax=[]  UdiffTsProdOutMin=[]  UdiffTsProdOutMax=[]  NTsProdOutMin=[]  NTsProdOutMax=[]  UintegralTsProdOutMin=[]  UintegralTsProdOutMax=[]  UngainTsProdOutMin=[]  UngainTsProdOutMax=[]  ClampingZeroOutDataTypeStr=Inherit: Inherit via back propagation  ClampingZeroOutMin=[]  ClampingZeroOutMax=[]  FilterDenConstantOutDataTypeStr=Inherit: Inherit via back propagation  FilterDenConstantOutMin=[]  FilterDenConstantOutMax=[]  PCopyOutDataTypeStr=Inherit: Inherit via back propagation  PCopyOutMin=[]  PCopyOutMax=[]  NCopyOutDataTypeStr=Inherit: Inherit via back propagation  NCopyOutMin=[]  NCopyOutMax=[]  IntegratorContinuousStateAttributes=''  IntegratorStateMustResolveToSignalObject=off  IntegratorRTWStateStorageClass=Auto  FilterContinuousStateAttributes=''  FilterStateMustResolveToSignalObject=off  FilterRTWStateStorageClass=Auto  ParallelPVariant=InternalParameters  IdealPVariant=Disabled  IVariant=InternalParameters  DVariant=Disabled  IntegratorVariant=Discrete  SatVariant=Enabled  AWVariant=Passthrough  PCopyVariant=Disabled  TRVariant=Disabled  FdbkBlocksVariant=Forward  IdealPFdbkVariant=Disabled  SatFdbkVariant=Disabled  DerivativeFilterVariant=Disabled  NVariant=Disabled  NCopyVariant=Disabled_SignalSpec  FilterICVariant=Disabled  IntegratorICVariant=InternalICs  ExternalResetVariant=Disabled  TRSumVariant=Passthrough  SumFdbkVariant=Disabled  SumVariant=Sum_PI  TsampFilterVariant=InternalTs  TsampNgainVariant=Passthrough  TsampIntegralVariant=Disabled_SignalSpec  ExternalSaturationOutDataTypeStr=Inherit: Same as second input  DerivativeSourceVariant=Disabled  PreIntVariant=InternalPreInt
  PWM Generator : eePwmGenerator/PWM Generator  CarrCount=Up  Tper=Ts  Tdelay=0  Ts=0
  Sum1 : Sum  Inputs=|+-
  PWM1 : Outport
  PWM2 : Outport  Port=2
  wires:
  Data Type Conversion2/1 -> NOT1/1
  NOT1/1 -> Data Type Conversion1/1
  Current control/1 -> Sum1/1
  Sum1/1 -> PID Controller/1
  Ibatt/1 -> Sum1/2
  Data Type Conversion1/1 -> PWM2/1
  PID Controller/1 -> PWM Generator/1
  PWM Generator/1 -> PWM1/1, Data Type Conversion2/1

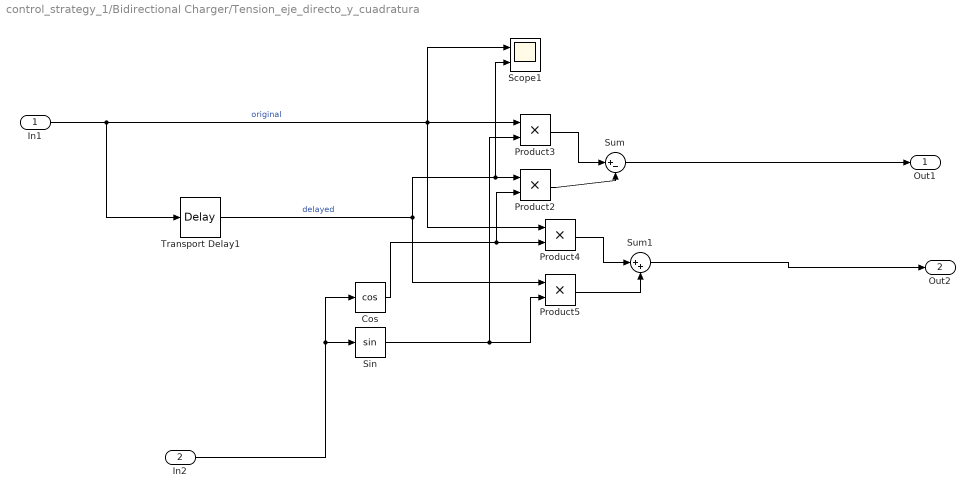
== system control_strategy_1/Bidirectional Charger/Tension_eje_directo_y_cuadratura ==
  In1 : Inport
  In2 : Inport  Port=2
  Cos : Trigonometry  Operator=cos
  Product{2..5} (4 alike) : Product
  Scope1 : Scope  NumInputPorts=2
  Sin : Trigonometry
  Sum : Sum  Inputs=|+-
  Sum1 : Sum  Inputs=|++
  Transport Delay1 : TransportDelay  DelayTime=0.25/60
  Out1 : Outport
  Out2 : Outport  Port=2
  wires:
  Product2/1 -> Sum/2
  Cos/1 -> Product4/2, Product2/2
  Transport Delay1/1 -> Scope1/2, Product2/1, Product5/1  "delayed"
  In1/1 -> Transport Delay1/1, Product4/1, Product3/1, Scope1/1  "original"
  Sum1/1 -> Out2/1
  Sum/1 -> Out1/1
  Sin/1 -> Product3/2, Product5/2
  Product5/1 -> Sum1/2
  Product3/1 -> Sum/1
  Product4/1 -> Sum1/1
  In2/1 -> Cos/1, Sin/1

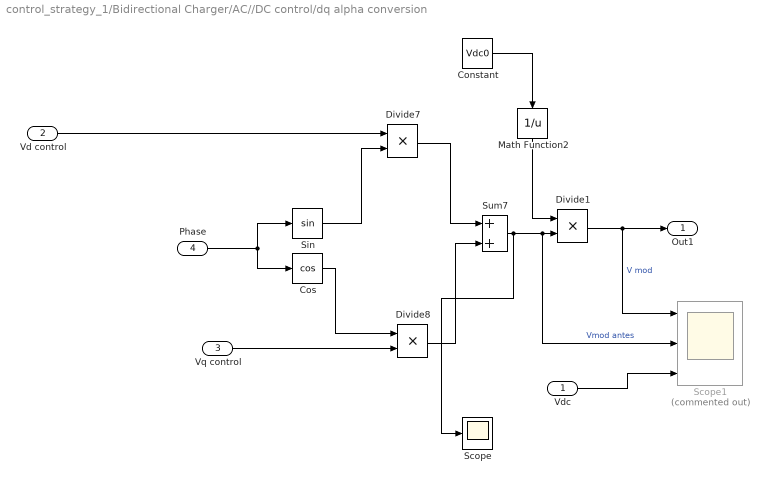
== system control_strategy_1/Bidirectional Charger/AC//DC control/dq alpha conversion ==
  Vdc : Inport
  Vd control : Inport  Port=2
  Vq control : Inport  Port=3
  Phase : Inport  Port=4
  Constant : Constant  Value=Vdc0
  Cos : Trigonometry  Operator=cos
  Divide1 : Product  Inputs=**
  Divide7 : Product  Inputs=**
  Divide8 : Product  Inputs=**
  Math Function2 : Math  Operator=reciprocal
  Scope : Scope
  Scope1 : Scope  Commented=on  NumInputPorts=3
  Sin : Trigonometry
  Sum7 : Sum
  Out1 : Outport
  wires:
  Cos/1 -> Divide8/1
  Sin/1 -> Divide7/2
  Vd control/1 -> Divide7/1
  Divide8/1 -> Sum7/2
  Divide7/1 -> Sum7/1
  Phase/1 -> Cos/1, Sin/1
  Vq control/1 -> Divide8/2
  Sum7/1 -> Scope/1, Scope1/2, Divide1/2  "Vmod antes"
  Divide1/1 -> Scope1/1, Out1/1  "V mod"
  Vdc/1 -> Scope1/3
  Math Function2/1 -> Divide1/1
  Constant/1 -> Math Function2/1
